simulink model "PD_driver_model"  (R2024b)
settings: Solver=FixedStepAuto  StartTime=0.0  StopTime=10.0  FixedStep=0.01  RelTol=1e-3
values from neighbouring files (symbols this model uses):
  A = [0, 1, u0, 0 ... (first row only)    [PD_driver_model.m]    (also in PD_driver_model_parameter.m)
  B = [0 ... (first row only)    [PD_driver_model.m]    (also in PD_driver_model_parameter.m)
  C = eye(4)    [PD_driver_model.m]    (also in PD_driver_model_parameter.m)
  D = zeros(4,1)    [PD_driver_model.m]    (also in PD_driver_model_parameter.m)
  Kd = Kd_values(i)    [PD_driver_model.m]    (also in PD_driver_model_parameter.m)
  Kp = 1    [PD_driver_model.m]    (also in PD_driver_model_parameter.m)
  N = 100    [PD_driver_model.m]    (also in PD_driver_model_parameter.m; Pure_Pursuit_Model.m)
settings Model: Creator=Corey  LastModifiedBy=Corey

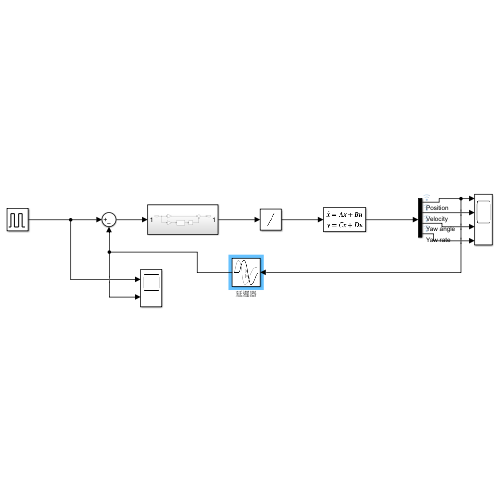
[thumbnail: Simulink's stored preview of the top-level diagram]
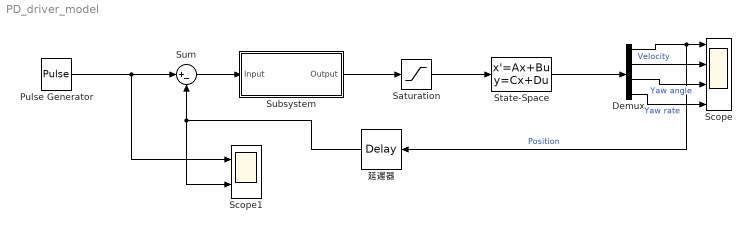
== system PD_driver_model ==
  Demux : Demux
  Pulse Generator : DiscretePulseGenerator  PulseType=Time based  Amplitude=4  Period=7  PulseWidth=50  PhaseDelay=0.5
  Saturation : Saturate  UpperLimit=48.7  LowerLimit=-48.7
  Scope : Scope  NumInputPorts=4
  Scope1 : Scope  NumInputPorts=2
  State-Space : StateSpace  A=A  B=B  C=C  D=D  InitialCondition=0
  Subsystem : Subsystem
  Sum : Sum  Inputs=|+-
  延遲器 : TransportDelay  DelayTime=0.03
  wires:
  Pulse Generator/1 -> Scope1/1, Sum/1
  Sum/1 -> Subsystem/1(Input)
  Subsystem/1(Output) -> Saturation/1
  Saturation/1 -> State-Space/1
  State-Space/1 -> Demux/1
  Demux/1 -> 延遲器/1, Scope/1  "Position"
  Demux/4 -> Scope/4  "Yaw rate"
  Demux/3 -> Scope/3  "Yaw angle"
  Demux/2 -> Scope/2  "Velocity"
  延遲器/1 -> Scope1/2, Sum/2

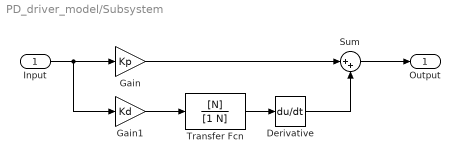
== system PD_driver_model/Subsystem ==
  Input : Inport
  Derivative : Derivative
  Gain : Gain  Gain=Kp
  Gain1 : Gain  Gain=Kd
  Sum : Sum  Inputs=|++
  Transfer Fcn : TransferFcn  Numerator=[N]  Denominator=[1 N]
  Output : Outport
  wires:
  Input/1 -> Gain1/1, Gain/1
  Transfer Fcn/1 -> Derivative/1
  Sum/1 -> Output/1
  Gain/1 -> Sum/1
  Derivative/1 -> Sum/2
  Gain1/1 -> Transfer Fcn/1
